simulink model "Bands5"  (R2018a)
settings: Solver=VariableStepAuto  StartTime=0.0  StopTime=0.01  RelTol=1e-3
undefined symbols (not defined in the file): fdesignblkfcn, G1, G2, G3, G4, G5, gcbh, get, T
libraries: dspsrcs4 x1, dspxfrm3 x1, dspobslib x1
(part 1 of 2)
settings Model: Creator=Daniel  LastModifiedBy=Daniel

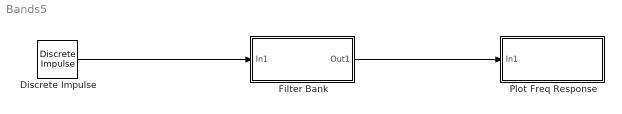
== system Bands5 ==
  Discrete Impulse : dspsrcs4/Discrete  Impulse  Delay=0  SampleTime=T  FrameSample=128  OutputFrames=off  dataType=double  isSigned=on  wordLen=16  udDataType=sfix(16)  fracBitsMode=Best precision  numFracBits=15  OutDataTypeStr=double  LastOutDataTypeStr=double
  "Filter Bank " : Subsystem
  Plot Freq Response : Subsystem
  wires:
  Discrete Impulse/1 -> "Filter Bank "/1(In1)
  "Filter Bank "/1(Out1) -> Plot Freq Response/1(In1)

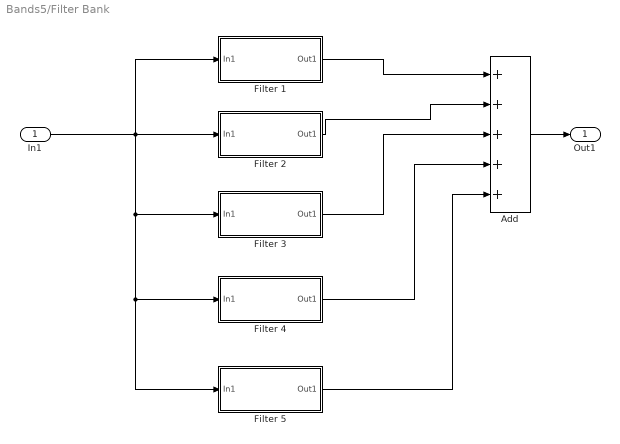
== system Bands5/Filter Bank  ==
  In1 : Inport
  Add : Sum  Inputs=+++++
  Filter 1 : Subsystem
  Filter 2 : Subsystem
  Filter 3 : Subsystem
  Filter 4 : Subsystem
  Filter 5 : Subsystem
  Out1 : Outport
  wires:
  In1/1 -> Filter 3/1(In1), Filter 5/1(In1), Filter 4/1(In1), Filter 1/1(In1), Filter 2/1(In1)
  Add/1 -> Out1/1
  Filter 1/1(Out1) -> Add/1
  Filter 2/1(Out1) -> Add/2
  Filter 3/1(Out1) -> Add/3
  Filter 4/1(Out1) -> Add/4
  Filter 5/1(Out1) -> Add/5

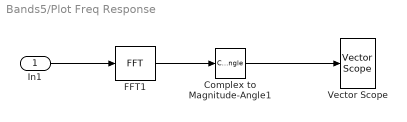
== system Bands5/Plot Freq Response ==
  In1 : Inport
  Complex to Magnitude-Angle1 : ComplexToMagnitudeAngle  Output=Magnitude
  FFT1 : dspxfrm3/FFT  FFTImplementation=Auto  CompMethod=Table lookup  TableOpt=NEW  TableOptActive=Speed  BitRevOrder=off  Normalize=off  InheritFFTLength=on  FFTLength=64  WrapInput=on  roundingMode=Floor  overflowMode=off  firstCoeffDataTypeStr=Inherit: Same word length as input  firstCoeffLastDataTypeStr=Inherit: Same word length as input  outputMin=[]  outputMax=[]
  Vector Scope : dspobslib/Vector Scope  ScopeProperties=off  Domain=Frequency  HorizSpan=1  DisplayProperties=off  AxisGrid=on  Memory=off  FrameNumber=off  AxisLegend=off  AxisZoom=off  OpenScopeAtSimStart=on  OpenScopeImmediately=off  FigPos=get(0,'defaultfigureposition')  AxisProperties=on  XUnits=Hertz  XRange=[0...Fs/2]  InheritXIncr=on  XIncr=1  XLabel=Samples  XLimit=Auto  XMin=0  XMax=1  XStart=0  YUnits=dB  YLabel=|Magnitude (dB)|  LineProperties=off  XAxisParamsVer=6.9
      settings: SourceProductName=DSP System Toolbox  SourceProductBaseCode=DS  YMin=0.0723692553519949  YMax=69.3188381671759
  wires:
  In1/1 -> FFT1/1
  FFT1/1 -> Complex to Magnitude-Angle1/1
  Complex to Magnitude-Angle1/1 -> Vector Scope/1

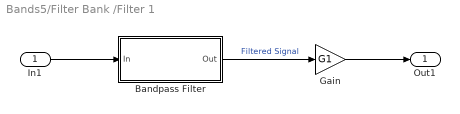
== system Bands5/Filter Bank /Filter 1 ==
  In1 : Inport
  Bandpass Filter : Subsystem  DialogController=fdesignblkfcn  InitFcn=fdesignblkfcn(gcbh, {'InitFcn'});  mask(Bandpass Filter){}
      mask help: Design a bandpass filter
      settings: CopyFcn=fdesignblkfcn(gcbh, {'CopyFcn'});
      mask Help: helpview(mapfilelocation('dsp'), 'dspbandpassfilter');
      mask Display: disp('Bandpass');
  Gain : Gain  Gain=G1
  Out1 : Outport
  wires:
  Bandpass Filter/1(Out) -> Gain/1  "Filtered Signal"
  In1/1 -> Bandpass Filter/1(In)
  Gain/1 -> Out1/1

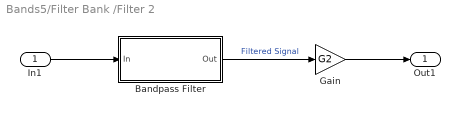
== system Bands5/Filter Bank /Filter 2 ==
  In1 : Inport
  Bandpass Filter : Subsystem  DialogController=fdesignblkfcn  InitFcn=fdesignblkfcn(gcbh, {'InitFcn'});  mask(Bandpass Filter){}
      mask help: Design a bandpass filter
      settings: CopyFcn=fdesignblkfcn(gcbh, {'CopyFcn'});
      mask Help: helpview(mapfilelocation('dsp'), 'dspbandpassfilter');
      mask Display: disp('Bandpass');
  Gain : Gain  Gain=G2
  Out1 : Outport
  wires:
  Bandpass Filter/1(Out) -> Gain/1  "Filtered Signal"
  In1/1 -> Bandpass Filter/1(In)
  Gain/1 -> Out1/1

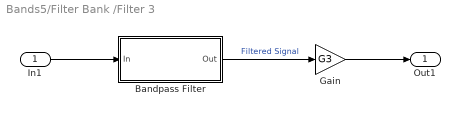
== system Bands5/Filter Bank /Filter 3 ==
  In1 : Inport
  Bandpass Filter : Subsystem  DialogController=fdesignblkfcn  InitFcn=fdesignblkfcn(gcbh, {'InitFcn'});  mask(Bandpass Filter){}
      mask help: Design a bandpass filter
      settings: CopyFcn=fdesignblkfcn(gcbh, {'CopyFcn'});
      mask Help: helpview(mapfilelocation('dsp'), 'dspbandpassfilter');
      mask Display: disp('Bandpass');
  Gain : Gain  Gain=G3
  Out1 : Outport
  wires:
  Bandpass Filter/1(Out) -> Gain/1  "Filtered Signal"
  In1/1 -> Bandpass Filter/1(In)
  Gain/1 -> Out1/1

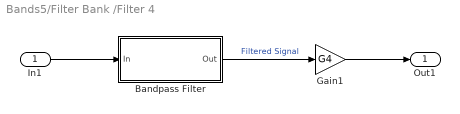
== system Bands5/Filter Bank /Filter 4 ==
  In1 : Inport
  Bandpass Filter : Subsystem  DialogController=fdesignblkfcn  InitFcn=fdesignblkfcn(gcbh, {'InitFcn'});  mask(Bandpass Filter){}
      mask help: Design a bandpass filter
      settings: CopyFcn=fdesignblkfcn(gcbh, {'CopyFcn'});
      mask Help: helpview(mapfilelocation('dsp'), 'dspbandpassfilter');
      mask Display: disp('Bandpass');
  Gain1 : Gain  Gain=G4
  Out1 : Outport
  wires:
  Bandpass Filter/1(Out) -> Gain1/1  "Filtered Signal"
  In1/1 -> Bandpass Filter/1(In)
  Gain1/1 -> Out1/1

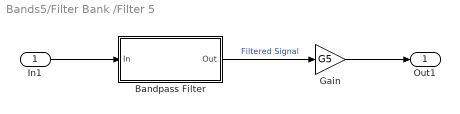
== system Bands5/Filter Bank /Filter 5 ==
  In1 : Inport
  Bandpass Filter : Subsystem  DialogController=fdesignblkfcn  InitFcn=fdesignblkfcn(gcbh, {'InitFcn'});  mask(Bandpass Filter){}
      mask help: Design a bandpass filter
      settings: CopyFcn=fdesignblkfcn(gcbh, {'CopyFcn'});
      mask Help: helpview(mapfilelocation('dsp'), 'dspbandpassfilter');
      mask Display: disp('Bandpass');
  Gain : Gain  Gain=G5
  Out1 : Outport
  wires:
  Bandpass Filter/1(Out) -> Gain/1  "Filtered Signal"
  In1/1 -> Bandpass Filter/1(In)
  Gain/1 -> Out1/1

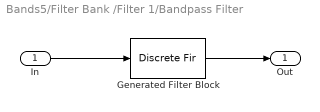
== system Bands5/Filter Bank /Filter 1/Bandpass Filter ==
  In : Inport
  Generated Filter Block : DiscreteFir  Tag=BlockMethodSubSystem  Coefficients=[-5.77791513980180748e-06 -2.30256955635310182e-05 -6.38284218907895964e-05 -0.000143375593985590858 -0.000278145909139618718 -0.000481101934859365864 -0.000755196488884121741 -0.00108642628461800704 -0.00143854197183239342 -0.0017518709474253079 -0.00194835989933904398 -0.00194372147515506919 -0.00166565575835332961 -0.00107488839069125102 -0.000183935151855407324 0.000932280857165333461 0.00213896288450997557 0.00325954827122383085 0.00410785031278295635 0.00452838880947028111 0.00443558337771372303 0.00384117533317485408 0.00286081836865718746 0.00169530027589830622 0.000588420544955621625 -0.000229636113125827413 -0.000599399499385923806 -0.000474123376884272719 6.60689785710101313e-05 0.000833714465226449426 0.00158370886128744791 0.00208060087726691942 0.00216488785307706027 0.00179890415989339349 0.00107798405245027105 0.000202356625653856196 -0.000582961988907336774 -0.00106283193805288253 -0.00111853054369610936 -0.00076519028308754105 -0.000147591717392950197 0.000505349439291061958 0.000953776076753570226 0.0010247228756057737 0.000669321045980362703 -1.99044420116749061e-05 -0.000838290082886334622 -0.00153619096711940344 -0.00190244313326051176 -0.00183639332849219478 -0.00138380466775325046 -0.000723496787874088466 -0.000108032944087852069 0.000222350497100262006 0.000123561348303465014 -0.000399926375045480884 -0.00119318444331612331 -0.00200159122221255613 -0.00255799392080699548 -0.00267670508440433306 -0.00232137811698231123 -0.00162192388437988567 -0.000832835469935237728 -0.000245834975920229508 -8.64709325591614614e-05 -0.000431064425303962937 -0.00117444191217202501 -0.00206179914741024765 -0.00277551664651013493 -0.00304764726407884875 -0.00275845543312811924 -0.00198491633972631585 -0.000979777679992968435 -8.61521300199152287e-05 0.000383853140290202062 0.00026380307606863263 -0.000401021934110337523 -0.00136212101383828663 -0.00225065207083287094 -0.00270745089445643874 -0.00251466309413073304 -0.00168101498438270706 -0.000447702837026988211 0.000790486342697706984 0.00162344712193536814 0.00177526480167162332 0.00121067929111964541 0.000157705926689365823 -0.000965383556067175809 -0.00169595526211921161 -0.00169531515172922833 -0.000878580976744386009 0.000543208636278050424 0.00212796344029402961 0.00335512469331679473 0.00381362375718750229 0.00335760383878252414 0.00217121256638813827 0.000714673918131669521 -0.000433669983065560133 -0.000785710222150447788 -0.000127765860330874935 0.0013883165590080277 0.0032848390829559003 0.00491986062910061521 0.00571655120272199398 0.00537871067913498358 0.00401232337361462355 0.0021040851331923468 0.00035839454516120654 -0.000553405466736302362 -0.000242926784184890199 0.00123854879981014749 0.0033986825258123703 0.00546566567621694678 0.00666059884493746743 0.0064851491490752599 0.00491888529403687949 0.00244911988063640498 -8.56625982827145154e-05 -0.00178973497146761714 -0.00203927635993856942 -0.000726709519361510366 0.00167423680940069356 0.00425552488896043576 0.00598987900201242499 0.00610567308360630313 0.00438592244214419235 0.00127695363579346209 -0.00224308362068644396 -0.0049994734505940993 -0.00604641482104468185 -0.00502999231838805426 -0.00235104766600972501 0.00094294448897309631 0.0035115557329951138 0.00420313763533652039 0.00249344121854316739 -0.00128353332889900927 -0.00600957629758990322 -0.0101512732835694446 -0.0123046600511932495 -0.0117245233520481412 -0.00864178518080495686 -0.00423878902780961981 -0.000270441805133744243 0.00155118637875221402 0.000196801395910227266 -0.00425016897109149836 -0.0105462069613504687 -0.0166664446020806899 -0.0204996777857504378 -0.0206263795403122396 -0.0168996767163211992 -0.010601162378508118 -0.00408180888581802671 2.09527177704848383e-05 -0.000262129445383532732 -0.00544000101614785375 -0.0142341067369937905 -0.0238759605106738763 -0.0309784921106219351 -0.0327206085740719202 -0.0279498577277856597 -0.0178011871146914781 -0.00556248662553401278 0.00424551481337098139 0.00733980016805927098 ...(+4529 chars)]  InputProcessing=Columns as channels (frame based)
  Out : Outport
  wires:
  In/1 -> Generated Filter Block/1
  Generated Filter Block/1 -> Out/1

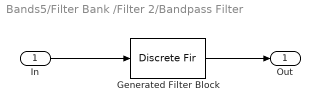
== system Bands5/Filter Bank /Filter 2/Bandpass Filter ==
  In : Inport
  Generated Filter Block : DiscreteFir  Tag=BlockMethodSubSystem  Coefficients=[-1.01953730652812796e-06 -4.59016410911419173e-06 -9.97669851388357789e-06 -1.08684869862469484e-05 3.60880799128958145e-06 3.73066045286563801e-05 7.12499280154968814e-05 6.16683292559652181e-05 -2.89163720499818928e-05 -0.000177733177488918488 -0.00027349015637737333 -0.000171192050764152888 0.000172046678081759605 0.000579275695689933259 0.000697915336458294834 0.000254775781151083541 -0.000631087834129832165 -0.00137140696253060723 -0.0012552755379029194 -5.81620667031764463e-05 0.00157475233456663742 0.00241672281878529266 0.00156626711803391086 -0.000684865990743256962 -0.00282415904973133116 -0.00315123922725677776 -0.00116703608508109211 0.00184367484869553963 0.00366646113060153283 0.00288279851769542971 6.09388817674600921e-05 -0.00265176266447713672 -0.00326141421620010146 -0.00152774842386365099 0.000948284938161425475 0.00219504451764179678 0.00154750301899494232 2.79801012009287235e-05 -0.000822391284707145453 -0.000452122434778858971 0.000322308375594950532 0.000355474155689936466 -0.000517964065941165278 -0.00129017571892501019 -0.000896375577618645984 0.000555521581637403506 0.00177448716218999336 0.001555242312451808 2.6350971810282376e-05 -0.00143351133751475047 -0.00154925236957868849 -0.00038492670495464973 0.000803816493321446142 0.000912278927583006914 8.94426637175626692e-05 -0.000547272308792595892 -0.000223698253382703693 0.000617485549233783861 0.000845536413463317325 -2.28003636875703839e-05 -0.00118609259956138245 -0.00136973223328524922 -0.000228739908099136001 0.00120472793360400102 0.00155980117818894102 0.000553012412897382921 -0.000741823411456300416 -0.0010706491724502738 -0.00032674647695879076 0.000428458363933233047 0.000248160494626968706 -0.000581141753760856003 -0.000872856933421154802 3.37204101876124689e-05 0.00138578559279310264 0.0017364701982928402 0.000532725962747075915 -0.00119507224250884584 -0.00186034205605397642 -0.000975036918446559454 0.000386908907386388347 0.000829409763041829293 0.00018094793241856517 -0.000402258842387320716 0.000109611460438225326 0.00129323520233204023 0.00165396120101479489 0.000355011598231368272 -0.001664746448441196 -0.00253548142256586817 -0.00141741444741097164 0.000584457764366390093 0.00160495427274504076 0.00100961735869166142 -3.39939545841485549e-05 -4.10377999868213959e-05 0.000967027123277885048 0.00144211564944913629 0.000181074649153619972 -0.00205260682211593501 -0.00311674093000307911 -0.00176624352526845896 0.000900009624799059504 0.00251224497832014653 0.00190594666313819859 0.000257111376404983976 -0.000399028915002676602 0.00042916283872559399 0.0011494134346434167 7.97876444765995832e-05 -0.00231502277681081437 -0.00362996041416430203 -0.00211039735325596481 0.00124145739951006594 0.00351844238001847165 0.0029076509579743573 0.000536103664258280122 -0.000922200939525845225 -0.000312431090997954998 0.000774342214546080033 5.92621269190715485e-05 -0.00244912665589219151 -0.00410632548713289053 -0.00251376448327567809 0.00155690664661633561 0.00463261313583291853 0.00408631632231015295 0.00088460175995070387 -0.00157713908612968972 -0.00128409950803707999 0.00026741345476661313 8.49732657066669021e-05 -0.00247320939186240416 -0.00456982132562619523 -0.00300659797367353564 0.0018456133792604378 0.00591564279559936464 0.00554261819590349571 0.00137171039499172373 -0.00238234283909111947 -0.00257510744291277599 -0.00045800100653825527 0.000127247211195181416 -0.00237536079793331445 -0.00501937579002808415 -0.00361161846694831468 0.00211282117552093066 0.00745326931732167089 0.00741457898485456922 0.00208292113955139404 -0.00338636660371552248 -0.00433676058684146371 -0.00153849218295913463 0.00014755673709161994 -0.00212583536705472165 -0.00544419530907839545 -0.00435621861900075454 0.00238019768909355101 0.00940004294210150179 0.00993392460484745186 0.0031446943107484417 -0.00470096411642826565 -0.00685000452601994183 -0.00320944172757841499 9.63793847029612661e-05 -0.00165942978307664652 -0.00583156476883985638 ...(+5974 chars)]  InputProcessing=Columns as channels (frame based)
  Out : Outport
  wires:
  In/1 -> Generated Filter Block/1
  Generated Filter Block/1 -> Out/1

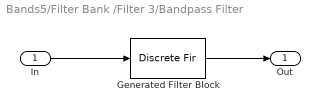
== system Bands5/Filter Bank /Filter 3/Bandpass Filter ==
  In : Inport
  Generated Filter Block : DiscreteFir  Tag=BlockMethodSubSystem  Coefficients=[-2.97500473341678406e-07 -6.68213225468835726e-07 7.378945868859321e-07 3.41239363423057309e-06 3.99894149735694521e-07 -9.87066438788385758e-06 -8.01732041175085057e-06 1.91276341772062409e-05 3.04469006129042364e-05 -2.32737598044607242e-05 -7.58871605933033179e-05 3.4933442359758795e-06 0.00014398371428579469 6.86952026074883414e-05 -0.000214775671605393399 -0.000221062237349536162 0.000241681128312557403 0.000461306158602609918 -0.000156882011212849232 -0.00075596132771586571 -0.00010613625426800959 0.00102036685359926851 0.000577361936624377209 -0.00113173554029384529 -0.00121711871711526875 0.00096802574508561578 0.00190436229478183451 -0.000460971183794997954 -0.0024595836254475271 -0.000359685377255956667 0.00269988741436763199 0.0013540316998794271 -0.00250672882173458463 -0.00230263319945342611 0.00187830854497910435 0.00297155165332716516 -0.000944006695037596542 -0.00318817398864531176 -6.59044367149521357e-05 0.00290088223653001305 0.00088516301304339439 -0.00220341012823266043 -0.00129123285902076317 0.00131663110220992343 0.00117846092746097184 -0.000529944028397169565 -0.000604706621815984764 0.000111563579725621514 -0.000207906066834222697 -0.000207335458507347927 0.000933409850300440254 0.000762870985515828686 -0.00126181669402816807 -0.00151386143552257051 0.00104361134183662092 0.00207636449919603892 -0.000390407845646164697 -0.00212316371626751314 -0.000341640640435088251 0.00157038139324981296 0.000712559319793888181 -0.000662323404317629542 -0.000443253454561907923 -0.000126508754434243893 -0.000392297195869484262 0.000351966685301804885 0.00136582220556119441 0.000115123097036115419 -0.00192417592763023128 -0.000968221511532946981 0.00173533057147470891 0.00161984153762470464 -0.000931109236469018471 -0.00156791681890522719 6.0984073436969597e-05 0.000746376703858946588 0.000250423556904685342 0.000391926212560206376 0.000265424707721756089 -0.00115236710173199377 -0.00130263517316861824 0.00107495598291224969 0.00215812778557828919 -0.000281244150950700608 -0.00221388942117005686 -0.000577853102901858284 0.00139445243261013762 0.000770956024177332604 -0.000254262736246708672 -2.8025579593060378e-05 -0.000402248499595154487 -0.00122870952812717234 0.000115651648453628949 0.00216575591875168031 0.000858997534800232327 -0.00215314129577264587 -0.00171073137212556978 0.00125986576891043379 0.00167352662264994207 -0.00023425625133975748 -0.000628927973452703582 -5.08151224953267623e-05 -0.000765279090678602542 -0.000715318239595004153 0.00155458630681420485 0.00200090579291738397 -0.00123295563802404374 -0.00280998639252266584 0.000172461760121011572 0.00245828154725876791 0.000630906183226965698 -0.00114495027888826041 -0.000334820122471947185 -0.000158944077277590795 -0.0010474211834201263 0.00046055350076066497 0.0026010153676597615 0.000438050480792901201 -0.00320320415190802421 -0.0017252252930357796 0.00243558462003039874 0.00218741640716129185 -0.000974933222401919782 -0.00119394988564121328 0.000100059519683670512 -0.000733202445039392997 -0.000660892712854700996 0.00227087224097561637 0.00233122752901629903 -0.00234249791065248682 -0.00379244076234459132 0.0010369222472754278 0.00376540462018891452 0.000383351870017709768 -0.0020890565886986269 -0.000462306770329679441 -5.86342023048393588e-05 -0.00122896604841000686 0.00105146393912847799 0.00364181379864103941 -0.000154577569167658595 -0.00501227757882437806 -0.00178291218795260486 0.00429026225074598342 0.00292094330573481036 -0.00208106347667299206 -0.0019109706357912544 0.000261757088850918425 -0.000914254940997310975 -0.000487333426763223289 0.00367677308949929463 0.0027603926209174524 -0.00441177024245775415 -0.00528366257303264624 0.00272283686809790711 0.00583022621509776597 -0.000245410361988895019 -0.00359833513532490214 -0.000578230383573367186 1.6791169467517143e-05 -0.00148176255576647794 0.00227557816896564388 0.00527659216490163237 -0.00156971990726416941 -0.00803367016978155137 -0.00137522095454260872 0.00756287266398526607 ...(+6828 chars)]  InputProcessing=Columns as channels (frame based)
  Out : Outport
  wires:
  In/1 -> Generated Filter Block/1
  Generated Filter Block/1 -> Out/1

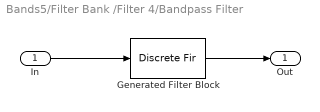
== system Bands5/Filter Bank /Filter 4/Bandpass Filter ==
  In : Inport
  Generated Filter Block : DiscreteFir  Tag=BlockMethodSubSystem  Coefficients=[1.35986709561009233e-07 -1.66961983060895873e-07 -4.7077530584272552e-07 1.26446726834643498e-06 1.1826702196979778e-07 -3.99342056850891331e-06 4.04078071244594997e-06 5.99285582339849786e-06 -1.59145867866124779e-05 2.33189358180343444e-06 3.21922358303557856e-05 -3.57251258390480858e-05 -3.04330269641059882e-05 9.6522527399939132e-05 -3.11287963869488093e-05 -0.000145201088825426501 0.000181261561125274715 8.88318946939344078e-05 -0.00037300639154456733 0.00016995009524050042 0.000441154329011706847 -0.000616923209915541454 -0.000159935324828326501 0.00102040477168909493 -0.000570033252843578603 -0.000972588862242522749 0.00151038615832298348 0.000152089970903371155 -0.00206459206645863425 0.001317839289271491 0.00159722014736567337 -0.00272673766874735341 3.57874865569260577e-05 0.00310699795722579929 -0.00216225070625789993 -0.00193174859622681581 0.00357005631872158889 -0.000337905938994981052 -0.00333563865107366258 0.0024116665535377055 0.00159883160455968529 -0.00307092037629337015 0.000437266079661024912 0.00214047625539721216 -0.00142151829588825756 -0.000652296035098371709 0.000970143378493510539 -4.64575247611137597e-05 3.44742818264756449e-05 -0.000502898986631040643 -0.000304336054198781037 0.00148521081236104935 -0.00060386934885010065 -0.00165707124696159698 0.00186809661374136922 0.000620110928686328248 -0.00225953976592784163 0.000766426268131039897 0.00142740488299650551 -0.0012847397835054578 -0.000269125868465581292 0.000646230044643726349 -3.04263671602194163e-05 0.000209850556818432405 -0.000721853613774392153 -0.000153969284362150908 0.0015281192254802073 -0.000879046821124028987 -0.00132420057430197337 0.00181761946204375907 0.000190014566306894025 -0.00167061397189139228 0.000730262083607253251 0.000670647562569265171 -0.000537297486276005955 -1.98755044403846137e-05 -0.000373650823857000472 0.000497090809921084897 0.000759625695085720419 -0.001531775765234674 9.25992824892191493e-06 0.00185754665117482095 -0.0011808886785489095 -0.00101726764175712214 0.00148950692448447577 -5.96947087473644012e-05 -0.000674261907318426555 0.000142080104954238329 -0.000169617492191517197 0.000809447059799040967 -0.000115523650976671411 -0.0015495980712197481 0.00132550239142735591 0.00103437139897214186 -0.00208862395760568177 0.000274653051420818261 0.00151670926947252631 -0.000914201039703968097 -0.00033507629166388349 0.000197490340772894909 5.48579817645800127e-05 0.000886314011872910775 -0.00111652453150173567 -0.000827281154018175082 0.0022766256876185836 -0.000529855192623547838 -0.0020816523277399487 0.00171101831411584718 0.000693692709466983519 -0.0013823486164315391 0.000219519031344598571 4.9749321601543872e-05 0.000488461301016914883 0.000472173575141465263 -0.00195084274782484192 0.000709862703766443249 0.0022633968989108238 -0.00236705676485632907 -0.000847391086225829284 0.00257674955083578121 -0.000722923120701708384 -0.00113309776217725448 0.000590026668075639845 -7.52305417708223196e-05 0.00102673696022835765 -0.000655463183834368527 -0.00196976176250583147 0.00264292239231096911 0.000778425391082819464 -0.00352572456486056245 0.00138433056510989857 0.00217743498305481443 -0.00203981827066716326 -0.000241354293842477741 0.000487491761850317043 0.000211979530727404893 0.00116643562724005 -0.00228111250134867098 -0.000521217727692229859 0.00392063538103809821 -0.00204188153683318224 -0.00294186619857437267 0.00364380938595635154 0.000343901420076233102 -0.00243647051995477155 0.000740733566360912959 6.38898105058627536e-05 0.00106495810570774677 0.000203621149056198124 -0.00346902334917079504 0.00242079695112165996 0.00319641665124928941 -0.00502959494995915482 -0.000152531931568350692 0.0044978379206802423 -0.00220924340873847802 -0.00151031695004860927 0.00108619632228874581 -3.31961843144192351e-05 0.00199040304903630406 -0.00217364548395669512 -0.00280090178773294849 0.00572122005298218283 -0.000298947670984078991 -0.00623071307454765681 0.00403393966279850039 0.00287832693448919182 ...(+7322 chars)]  InputProcessing=Columns as channels (frame based)
  Out : Outport
  wires:
  In/1 -> Generated Filter Block/1
  Generated Filter Block/1 -> Out/1
